simulink subsystem "pll_encoder"  (R2023b)
settings: Solver=VariableStepAuto  StartTime=0.0  StopTime=10.0  RelTol=1e-3
model mask{pole_1_Hz=-10, pole_2_Hz=-100}
  mask prompts: pole_1_Hz "Pole 1 (Hz)"; pole_2_Hz "Pole 2 (Hz)"
undefined symbols (not defined in the file): CTRL, DiscIntNeverNeededParam
settings Model: Creator=Nathan Petersen  LastModifiedBy=ericseverson

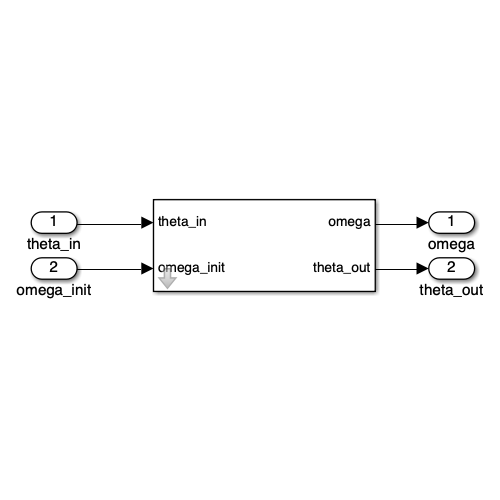
[thumbnail: Simulink's stored preview of the top-level diagram]
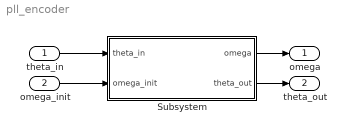
== system pll_encoder ==
  theta_in : Inport
  omega_init : Inport  Port=2
  Subsystem : Subsystem  mask{pole_1_Hz=-10, pole_2_Hz=-100}
      mask prompts: pole_1_Hz "Pole 1 (Hz)"; pole_2_Hz "Pole 2 (Hz)"
      mask DialogControl DescTextVar Prompt: Implements typical continuous-time PLL as approximate discrete-time version vased on backwards Euler integration. <br> <br> Tune by specifying the location of 2 poles in continuous-time left-half plane.
      mask DialogControl ParametersLabel Prompt: Parameters
  omega : Outport
  theta_out : Outport  Port=2
  wires:
  theta_in/1 -> Subsystem/1(theta_in)
  omega_init/1 -> Subsystem/2(omega_init)
  Subsystem/1(omega) -> omega/1
  Subsystem/2(theta_out) -> theta_out/1

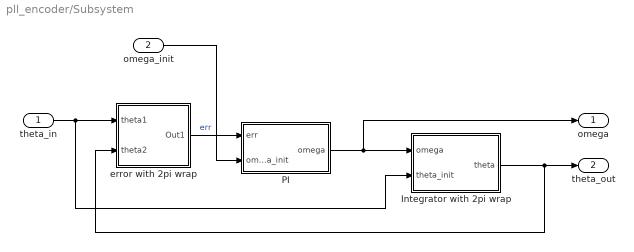
== system pll_encoder/Subsystem ==
  theta_in : Inport
  omega_init : Inport  Port=2
  Integrator with 2pi wrap : Subsystem
  PI : Subsystem
  error with 2pi wrap : Subsystem
  omega : Outport
  theta_out : Outport  Port=2
  wires:
  theta_in/1 -> error with 2pi wrap/1(theta1), Integrator with 2pi wrap/2(theta_init)
  omega_init/1 -> PI/2(omega_init)
  PI/1(omega) -> omega/1, Integrator with 2pi wrap/1(omega)
  error with 2pi wrap/1(Out1) -> PI/1(err)  "err"
  Integrator with 2pi wrap/1(theta) -> theta_out/1, error with 2pi wrap/2(theta2)

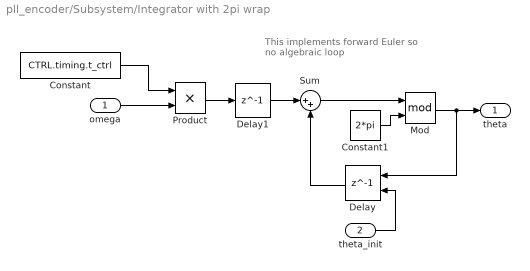
== system pll_encoder/Subsystem/Integrator with 2pi wrap ==
  note: This implements forward Euler so no algebraic loop
  omega : Inport
  theta_init : Inport  Port=2
  Constant : Constant  Value=CTRL.timing.t_ctrl
  Constant1 : Constant  Value=2*pi
  Delay : Delay  DelayLength=1  InitialConditionSource=Input port
      settings: InputPortMap=u0,p4
  Delay1 : Delay  DelayLength=1
  Mod : Math  Operator=mod
  Product : Product
  Sum : Sum  Inputs=|++
  theta : Outport
  wires:
  theta_init/1 -> Delay/2
  Delay1/1 -> Sum/1
  Mod/1 -> theta/1, Delay/1
  Sum/1 -> Mod/1
  Constant1/1 -> Mod/2
  Delay/1 -> Sum/2
  Product/1 -> Delay1/1
  Constant/1 -> Product/1
  omega/1 -> Product/2

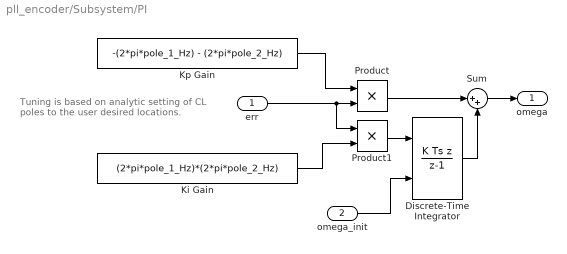
== system pll_encoder/Subsystem/PI ==
  note: Tuning is based on analytic setting of CL poles to the user desired locations.
  err : Inport
  omega_init : Inport  Port=2
  Discrete-Time Integrator : DiscreteIntegrator  IntegratorMethod=Integration: Backward Euler  InitialConditionSource=external  SampleTime=-1  ICPrevOutput=DiscIntNeverNeededParam  ICPrevScaledInput=DiscIntNeverNeededParam
  Ki Gain : Constant  Value=(2*pi*pole_1_Hz)*(2*pi*pole_2_Hz)
  Kp Gain : Constant  Value=-(2*pi*pole_1_Hz) - (2*pi*pole_2_Hz)
  Product : Product
  Product1 : Product
  Sum : Sum  Inputs=|++
  omega : Outport
  wires:
  omega_init/1 -> Discrete-Time Integrator/2
  Discrete-Time Integrator/1 -> Sum/2
  Product1/1 -> Discrete-Time Integrator/1
  Ki Gain/1 -> Product1/2
  Kp Gain/1 -> Product/1
  Product/1 -> Sum/1
  err/1 -> Product/2, Product1/1
  Sum/1 -> omega/1

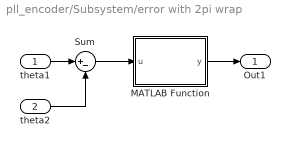
== system pll_encoder/Subsystem/error with 2pi wrap ==
  theta1 : Inport
  theta2 : Inport  Port=2
  MATLAB Function : MATLAB Function  TreatAsAtomicUnit=on
  Sum : Sum  Inputs=|+-
  Out1 : Outport
  wires:
  theta2/1 -> Sum/2
  MATLAB Function/1(y) -> Out1/1
  Sum/1 -> MATLAB Function/1(u)
  theta1/1 -> Sum/1

== matlab function pll_encoder/Subsystem/error with 2pi wrap/MATLAB Function ==
  data: u input; y output
function y = fcn(u)

y = u;

if y > pi
    y = y - 2*pi;
end

if y < -pi
    y = y + 2*pi;
end
